simulink model "Non_WindFarm"  (R2024a)
settings: Solver=ode45  StartTime=parSimulacio.ti  StopTime=200  MaxStep=parSimulacio.pas  RelTol=1e-6  AbsTol=1e-6  EnableMultiTasking=on
model workspace (MAT data in the model file):
  tt_vw = Simulink.Parameter
  tt_vw.Complexity = 'real'
  tt_vw.Dimensions = [0 0]
  tt_vw.DataType = 'auto'
values from neighbouring files (symbols this model uses):
  L = L'    [Lin_SignalGenerator.m]    (also in Non_ParameterInitialize.m; cal_QR.m = zeros(v, 1); parameters_windFarm2.m)
  nu = size(S, 1)    [Lin_SignalGenerator.m]    (also in Non_ParameterInitialize.m; parameters_windFarm2.m)
  S = zeros(v, v)    [cal_QR.m]
  w0 = [1 -0.00962521549583 0.0254779042049 -0.0160197396127 -0.0156056332727 0.0112137208272 0.0440607583301 -0.0193704893312 -0.0229464276306 -0.00247675309015 0.0285830611299]    [w0.mat]
undefined symbols (not defined in the file or in its folder): parControl, parConvertidor, parGenerador, parGrid, parMecanica, parSimulacio, windspeed
(part 1 of 40)
settings Model: SimulationMode=accelerator  Creator=adria  LastModifiedBy=hz1021
settings SolverCC: AlgebraicLoopSolver=TrustRegion
settings DataIOCC: LimitDataPoints=on  SaveFormat=Array  SignalLoggingSaveFormat=ModelDataLogs  SaveOutput=off  SaveTime=off  ReturnWorkspaceOutputs=off
settings OptimizationCC: ReuseModelBlockBuffer=off  InitFltsAndDblsToZero=on  LifeSpan=inf
settings DebuggingCC: SaveWithParameterizedLinksMsg=none  UnderspecifiedInitializationDetection=Classic  MergeDetectMultiDrivingBlocksExec=none  SignalResolutionControl=TryResolveAllWithWarning  SolverPrmCheckMsg=warning  FcnCallInpInsideContextMsg=warning  UnconnectedInputMsg=warning  UnconnectedOutputMsg=warning  UnconnectedLineMsg=warning  SFUnexpectedBacktrackingDiag=warning  SFNoUnconditionalDefaultTransitionDiag=warning  SFExecutionAtInitializationDiag=none  ArithmeticOperatorsInVariantConditions=warning
settings HardwareCC: ProdBitPerPointer=32  ProdBitPerSizeT=32  ProdBitPerPtrDiffT=32  ProdLargestAtomicFloat=None  ProdIntDivRoundTo=Undefined  ProdEndianess=Unspecified  ProdWordSize=32  ProdHWDeviceType=32-bit Generic
settings ModelReferenceCC: EnableRefExpFcnMdlSchedulingChecks=on  PropagateSignalLabelsOutOfModel=off
settings RTWCC: GPUComputeCapability=3.5  DLArmComputeVersion=19.05
settings CodeAppCC: StateflowObjectComments=on
settings GRTTargetCC: TargetFcnLib=ansi_tfl_tmw.mat  TargetLangStandard=C89/C90 (ANSI)  CombineOutputUpdateFcns=off  GRTInterface=on
settings ConfigComp: CovMetricSettings=dw  CovSaveCumulativeToWorkspaceVar=on  CovSaveSingleToWorkspaceVar=on

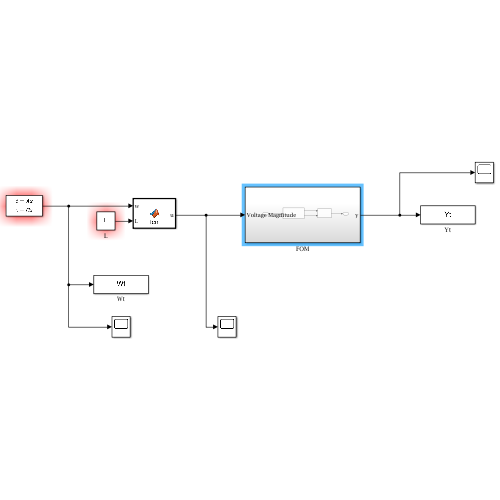
[thumbnail: Simulink's stored preview of the top-level diagram]
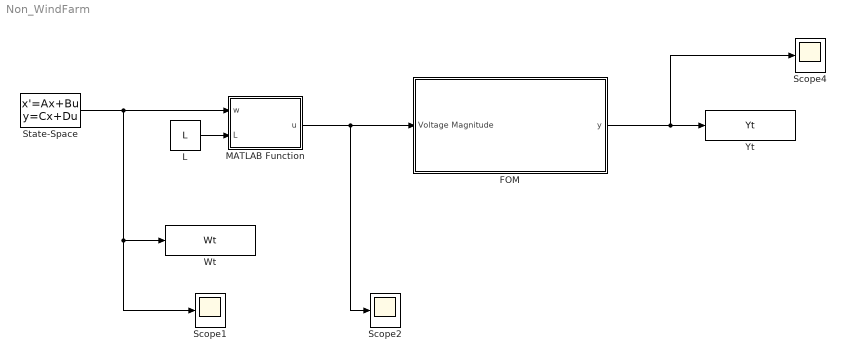
== system Non_WindFarm ==
  FOM : Subsystem
  L : Constant  Value=L
  MATLAB Function : MATLAB Function  TreatAsAtomicUnit=on
  Scope1 : Scope
  Scope2 : Scope
  Scope4 : Scope
  State-Space : StateSpace  A=S  B=[]  C=eye(nu)  D=[]  InitialCondition=w0  AbsoluteTolerance=1e-6
  Wt : ToWorkspace  VariableName=Wt  SaveFormat=Timeseries  SampleTime=-1
  Yt : ToWorkspace  VariableName=Yt  SaveFormat=Timeseries  SampleTime=-1
  wires:
  FOM/1(y) -> Yt/1, Scope4/1
  MATLAB Function/1(u) -> FOM/1(Voltage Magnitude), Scope2/1
  State-Space/1 -> Wt/1, Scope1/1, MATLAB Function/1(w)
  L/1 -> MATLAB Function/2(L)

== system Non_WindFarm/FOM ==
  Voltage Magnitude : Inport
  MATLAB Function2 : MATLAB Function  TreatAsAtomicUnit=on
  Wind Farm : Subsystem
  y : Outport
  wires:
  Wind Farm/2(Ic) -> MATLAB Function2/2(Ic)
  Voltage Magnitude/1 -> Wind Farm/1(Voltage Magnitude)
  Wind Farm/1(Vc) -> MATLAB Function2/1(Vc)
  MATLAB Function2/1(y) -> y/1

== system Non_WindFarm/FOM/Wind Farm ==
  Voltage Magnitude : Inport
  3phase2dq : Subsystem
  C at HV transf : Subsystem
  Gain1 : Gain  Gain=1/parGrid.WFtransf.rloss
  HV transf1 : Subsystem
  Scope1 : Scope
  Scope3 : Scope
  Subtract1 : Sum  Inputs=+-
  Wind Turbine Strings : Subsystem
  Vc : Outport
  Ic : Outport  Port=2
  wires:
  Subtract1/1 -> Scope3/1, Ic/1, C at HV transf/2(Itransf)
  3phase2dq/1(Vdq) -> HV transf1/1(Vin)
  HV transf1/1(Itransf) -> Subtract1/1
  C at HV transf/1(Vc) -> Wind Turbine Strings/1(V_in), Scope1/1, Vc/1, HV transf1/2(Vc), Gain1/1
  Gain1/1 -> Subtract1/2
  Voltage Magnitude/1 -> 3phase2dq/1(Voltage Magnitude)
  Wind Turbine Strings/1(I_out_tol) -> C at HV transf/1(Istrings)

== system Non_WindFarm/FOM/Wind Farm/3phase2dq ==
  Voltage Magnitude : Inport
  Clock2 : Clock
  Font trifasica asimetrica1 : Subsystem  mask{tempPar=parGrid.WFtransf}
      mask prompts: tempPar "Estruc. Parametres"
      mask init:
      | we=tempPar.f*2*pi;
      | A_D=tempPar.V_D*sqrt(2)/sqrt(3);
      | A_I=tempPar.V_I*sqrt(2)/sqrt(3);
      | phi_D=tempPar.phi_D;
      | phi_I=tempPar.phi_I;
      | tt_D=tempPar.tt_D;
      | tt_I=tempPar.tt_I;
      | tA_D=tempPar.tA_D;
      | tA_I=tempPar.tA_I;
  Product : Product
  Vdq : Outport
  wires:
  Product/1 -> Vdq/1
  Clock2/1 -> Font trifasica asimetrica1/1(t)
  Font trifasica asimetrica1/1(y) -> Product/1
  Voltage Magnitude/1 -> Product/2

== system Non_WindFarm/FOM/Wind Farm/C at HV transf ==
  note: Vc_cable
  Istrings : Inport
  Itransf : Inport  Port=2
  Add : Sum  Inputs=+-
  produce Vc_cable : StateSpace  A=[0,-100*pi;100*pi,0]  B=eye(2)/parGrid.WFtransf.Cfilt  C=eye(2)  D=zeros(2,2)  InitialCondition=sqrt(2)*66000/sqrt(3)*[1;0]
  Vc : Outport
  wires:
  produce Vc_cable/1 -> Vc/1
  Add/1 -> produce Vc_cable/1
  Itransf/1 -> Add/2
  Istrings/1 -> Add/1

== system Non_WindFarm/FOM/Wind Farm/HV transf1 ==
  Vin : Inport
  Vc : Inport  Port=2
  1/L_Cable : Gain  Gain=1/parGrid.WFtransf.L
  A : Constant  Value=[parGrid.WFtransf.r,100*pi*parGrid.WFtransf.L;-100*pi*parGrid.WFtransf.L,parGrid.WFtransf.r]
  Add : Sum  Inputs=+--
  Integrator : Integrator
  Product6 : Product  Multiplication=Matrix(*)
  Itransf : Outport
  wires:
  Integrator/1 -> Product6/2, Itransf/1
  Vc/1 -> Add/1
  Vin/1 -> Add/2
  A/1 -> Product6/1
  Product6/1 -> Add/3
  1/L_Cable/1 -> Integrator/1
  Add/1 -> 1/L_Cable/1

== system Non_WindFarm/FOM/Wind Farm/Wind Turbine Strings ==
  V_in : Inport
  Add : Sum  Inputs=6
  String1 : Subsystem
  String2 : Subsystem
  String3 : Subsystem  Commented=on
  String4 : Subsystem  Commented=on
  String5 : Subsystem  Commented=on
  String6 : Subsystem  Commented=on
  I_out_tol : Outport
  wires:
  V_in/1 -> String6/1(V_in), String5/1(V_in), String4/1(V_in), String3/1(V_in), String2/1(V_in), String1/1(V_in)
  String1/1(I_out) -> Add/1
  String2/1(I_out) -> Add/2
  Add/1 -> I_out_tol/1
  String3/1(I_out) -> Add/3
  String4/1(I_out) -> Add/4
  String5/1(I_out) -> Add/5
  String6/1(I_out) -> Add/6

== system Non_WindFarm/FOM/Wind Farm/3phase2dq/Font trifasica asimetrica1 ==
  t : Inport
  Clock : Clock
  Constant1 : Constant  Value=phi_D
  Constant2 : Constant  Value=phi_I
  Constant3 : Constant  Value=2*pi/3
  Constant4 : Constant  Value=2*pi/3
  Gain : Gain  Gain=we
  Gain1 : Gain  Gain=A_D
  Gain2 : Gain  Gain=A_I
  Mux : Mux  Inputs=3
  Mux1 : Mux  Inputs=3
  Park : Subsystem
  Product : Product  RndMeth=Zero
  Product1 : Product  RndMeth=Zero
  Product4 : Product  Multiplication=Matrix(*)  RndMeth=Zero
  Scope1 : Scope
  Sum{1,3,5..7} (5 alike) : Sum  Inputs=|++
  Sum2 : Sum  Inputs=|+-
  Sum4 : Sum  Inputs=|+-
  Trigonometric Function{1..6} (6 alike) : Trigonometry  Operator=cos
  directa : Lookup  InputValues=tt_D  Table=tA_D  SaturateOnIntegerOverflow=off
  inversa : Lookup  InputValues=tt_I  Table=tA_I  SaturateOnIntegerOverflow=off
  we : Gain  Gain=100*pi
  y : Outport
  wires:
  Sum3/1 -> Trigonometric Function2/1, Sum2/1, Sum1/1
  Sum2/1 -> Trigonometric Function1/1
  Sum1/1 -> Trigonometric Function3/1
  Constant4/1 -> Sum2/2, Sum1/2
  Trigonometric Function2/1 -> Mux/1
  Trigonometric Function1/1 -> Mux/2
  Trigonometric Function3/1 -> Mux/3
  Mux/1 -> Gain1/1
  t/1 -> Gain/1, directa/1, inversa/1
  Gain/1 -> Sum3/1, Sum6/1
  Constant1/1 -> Sum3/2
  Sum6/1 -> Trigonometric Function5/1, Sum5/1, Sum4/1
  Sum5/1 -> Trigonometric Function4/1
  Sum4/1 -> Trigonometric Function6/1
  Constant3/1 -> Sum4/2, Sum5/2
  Trigonometric Function5/1 -> Mux1/1
  Trigonometric Function4/1 -> Mux1/2
  Trigonometric Function6/1 -> Mux1/3
  Mux1/1 -> Gain2/1
  Constant2/1 -> Sum6/2
  Product/1 -> Sum7/1
  directa/1 -> Product/1
  inversa/1 -> Product1/1
  Gain1/1 -> Product/2
  Gain2/1 -> Product1/2
  Product1/1 -> Sum7/2
  Park/1(Tthetar) -> Scope1/1, Product4/1
  Clock/1 -> we/1
  we/1 -> Park/1(theta_r)
  Sum7/1 -> Product4/2
  Product4/1 -> y/1

== system Non_WindFarm/FOM/Wind Farm/Wind Turbine Strings/String1 ==
  V_in : Inport
  Constant : Constant  Value=0
  Scope : Scope
  WT1 : Subsystem
  WT10 : Subsystem
  WT2 : Subsystem
  WT3 : Subsystem
  WT4 : Subsystem
  WT5 : Subsystem
  WT6 : Subsystem
  WT7 : Subsystem
  WT8 : Subsystem
  WT9 : Subsystem
  I_out : Outport
  wires:
  WT10/1(V_out) -> Scope/1
  WT7/1(V_out) -> WT8/1(V_in)
  Constant/1 -> WT10/2(I_in)
  WT4/1(V_out) -> WT5/1(V_in)
  WT4/2(I_out) -> WT3/2(I_in)
  WT3/1(V_out) -> WT4/1(V_in)
  WT1/1(V_out) -> WT2/1(V_in)
  WT10/2(I_out) -> WT9/2(I_in)
  WT5/1(V_out) -> WT6/1(V_in)
  WT2/1(V_out) -> WT3/1(V_in)
  WT7/2(I_out) -> WT6/2(I_in)
  WT8/1(V_out) -> WT9/1(V_in)
  WT6/1(V_out) -> WT7/1(V_in)
  WT9/2(I_out) -> WT8/2(I_in)
  WT5/2(I_out) -> WT4/2(I_in)
  WT2/2(I_out) -> WT1/2(I_in)
  V_in/1 -> WT1/1(V_in)
  WT3/2(I_out) -> WT2/2(I_in)
  WT8/2(I_out) -> WT7/2(I_in)
  WT9/1(V_out) -> WT10/1(V_in)
  WT6/2(I_out) -> WT5/2(I_in)
  WT1/2(I_out) -> I_out/1

== system Non_WindFarm/FOM/Wind Farm/Wind Turbine Strings/String2 ==
  V_in : Inport
  Constant : Constant  Value=0
  Scope : Scope
  WT1 : Subsystem
  WT10 : Subsystem
  WT2 : Subsystem
  WT3 : Subsystem
  WT4 : Subsystem
  WT5 : Subsystem
  WT6 : Subsystem
  WT7 : Subsystem
  WT8 : Subsystem
  WT9 : Subsystem
  I_out : Outport
  wires:
  WT1/2(I_out) -> I_out/1
  WT6/2(I_out) -> WT5/2(I_in)
  WT9/1(V_out) -> WT10/1(V_in)
  WT8/2(I_out) -> WT7/2(I_in)
  WT3/2(I_out) -> WT2/2(I_in)
  V_in/1 -> WT1/1(V_in)
  WT2/2(I_out) -> WT1/2(I_in)
  WT5/2(I_out) -> WT4/2(I_in)
  WT9/2(I_out) -> WT8/2(I_in)
  WT6/1(V_out) -> WT7/1(V_in)
  WT8/1(V_out) -> WT9/1(V_in)
  WT7/2(I_out) -> WT6/2(I_in)
  WT2/1(V_out) -> WT3/1(V_in)
  WT5/1(V_out) -> WT6/1(V_in)
  WT10/2(I_out) -> WT9/2(I_in)
  WT1/1(V_out) -> WT2/1(V_in)
  WT3/1(V_out) -> WT4/1(V_in)
  WT4/2(I_out) -> WT3/2(I_in)
  WT4/1(V_out) -> WT5/1(V_in)
  Constant/1 -> WT10/2(I_in)
  WT7/1(V_out) -> WT8/1(V_in)
  WT10/1(V_out) -> Scope/1

== system Non_WindFarm/FOM/Wind Farm/Wind Turbine Strings/String3 ==
  V_in : Inport
  Constant : Constant  Value=0
  Scope : Scope
  WT1 : Subsystem
  WT10 : Subsystem
  WT2 : Subsystem
  WT3 : Subsystem
  WT4 : Subsystem
  WT5 : Subsystem
  WT6 : Subsystem
  WT7 : Subsystem
  WT8 : Subsystem
  WT9 : Subsystem
  I_out : Outport
  wires:
  WT1/2(I_out) -> I_out/1
  WT6/2(I_out) -> WT5/2(I_in)
  WT9/1(V_out) -> WT10/1(V_in)
  WT8/2(I_out) -> WT7/2(I_in)
  WT3/2(I_out) -> WT2/2(I_in)
  V_in/1 -> WT1/1(V_in)
  WT2/2(I_out) -> WT1/2(I_in)
  WT5/2(I_out) -> WT4/2(I_in)
  WT9/2(I_out) -> WT8/2(I_in)
  WT6/1(V_out) -> WT7/1(V_in)
  WT8/1(V_out) -> WT9/1(V_in)
  WT7/2(I_out) -> WT6/2(I_in)
  WT2/1(V_out) -> WT3/1(V_in)
  WT5/1(V_out) -> WT6/1(V_in)
  WT10/2(I_out) -> WT9/2(I_in)
  WT1/1(V_out) -> WT2/1(V_in)
  WT3/1(V_out) -> WT4/1(V_in)
  WT4/2(I_out) -> WT3/2(I_in)
  WT4/1(V_out) -> WT5/1(V_in)
  Constant/1 -> WT10/2(I_in)
  WT7/1(V_out) -> WT8/1(V_in)
  WT10/1(V_out) -> Scope/1

== system Non_WindFarm/FOM/Wind Farm/Wind Turbine Strings/String4 ==
  V_in : Inport
  Constant : Constant  Value=0
  Scope : Scope
  WT1 : Subsystem
  WT10 : Subsystem
  WT2 : Subsystem
  WT3 : Subsystem
  WT4 : Subsystem
  WT5 : Subsystem
  WT6 : Subsystem
  WT7 : Subsystem
  WT8 : Subsystem
  WT9 : Subsystem
  I_out : Outport
  wires:
  WT1/2(I_out) -> I_out/1
  WT6/2(I_out) -> WT5/2(I_in)
  WT9/1(V_out) -> WT10/1(V_in)
  WT8/2(I_out) -> WT7/2(I_in)
  WT3/2(I_out) -> WT2/2(I_in)
  V_in/1 -> WT1/1(V_in)
  WT2/2(I_out) -> WT1/2(I_in)
  WT5/2(I_out) -> WT4/2(I_in)
  WT9/2(I_out) -> WT8/2(I_in)
  WT6/1(V_out) -> WT7/1(V_in)
  WT8/1(V_out) -> WT9/1(V_in)
  WT7/2(I_out) -> WT6/2(I_in)
  WT2/1(V_out) -> WT3/1(V_in)
  WT5/1(V_out) -> WT6/1(V_in)
  WT10/2(I_out) -> WT9/2(I_in)
  WT1/1(V_out) -> WT2/1(V_in)
  WT3/1(V_out) -> WT4/1(V_in)
  WT4/2(I_out) -> WT3/2(I_in)
  WT4/1(V_out) -> WT5/1(V_in)
  Constant/1 -> WT10/2(I_in)
  WT7/1(V_out) -> WT8/1(V_in)
  WT10/1(V_out) -> Scope/1

== system Non_WindFarm/FOM/Wind Farm/Wind Turbine Strings/String5 ==
  V_in : Inport
  Constant : Constant  Value=0
  Scope : Scope
  WT1 : Subsystem
  WT10 : Subsystem
  WT2 : Subsystem
  WT3 : Subsystem
  WT4 : Subsystem
  WT5 : Subsystem
  WT6 : Subsystem
  WT7 : Subsystem
  WT8 : Subsystem
  WT9 : Subsystem
  I_out : Outport
  wires:
  WT1/2(I_out) -> I_out/1
  WT6/2(I_out) -> WT5/2(I_in)
  WT9/1(V_out) -> WT10/1(V_in)
  WT8/2(I_out) -> WT7/2(I_in)
  WT3/2(I_out) -> WT2/2(I_in)
  V_in/1 -> WT1/1(V_in)
  WT2/2(I_out) -> WT1/2(I_in)
  WT5/2(I_out) -> WT4/2(I_in)
  WT9/2(I_out) -> WT8/2(I_in)
  WT6/1(V_out) -> WT7/1(V_in)
  WT8/1(V_out) -> WT9/1(V_in)
  WT7/2(I_out) -> WT6/2(I_in)
  WT2/1(V_out) -> WT3/1(V_in)
  WT5/1(V_out) -> WT6/1(V_in)
  WT10/2(I_out) -> WT9/2(I_in)
  WT1/1(V_out) -> WT2/1(V_in)
  WT3/1(V_out) -> WT4/1(V_in)
  WT4/2(I_out) -> WT3/2(I_in)
  WT4/1(V_out) -> WT5/1(V_in)
  Constant/1 -> WT10/2(I_in)
  WT7/1(V_out) -> WT8/1(V_in)
  WT10/1(V_out) -> Scope/1

== system Non_WindFarm/FOM/Wind Farm/Wind Turbine Strings/String6 ==
  V_in : Inport
  Constant : Constant  Value=0
  Scope : Scope
  WT1 : Subsystem
  WT10 : Subsystem
  WT2 : Subsystem
  WT3 : Subsystem
  WT4 : Subsystem
  WT5 : Subsystem
  WT6 : Subsystem
  WT7 : Subsystem
  WT8 : Subsystem
  WT9 : Subsystem
  I_out : Outport
  wires:
  WT1/2(I_out) -> I_out/1
  WT6/2(I_out) -> WT5/2(I_in)
  WT9/1(V_out) -> WT10/1(V_in)
  WT8/2(I_out) -> WT7/2(I_in)
  WT3/2(I_out) -> WT2/2(I_in)
  V_in/1 -> WT1/1(V_in)
  WT2/2(I_out) -> WT1/2(I_in)
  WT5/2(I_out) -> WT4/2(I_in)
  WT9/2(I_out) -> WT8/2(I_in)
  WT6/1(V_out) -> WT7/1(V_in)
  WT8/1(V_out) -> WT9/1(V_in)
  WT7/2(I_out) -> WT6/2(I_in)
  WT2/1(V_out) -> WT3/1(V_in)
  WT5/1(V_out) -> WT6/1(V_in)
  WT10/2(I_out) -> WT9/2(I_in)
  WT1/1(V_out) -> WT2/1(V_in)
  WT3/1(V_out) -> WT4/1(V_in)
  WT4/2(I_out) -> WT3/2(I_in)
  WT4/1(V_out) -> WT5/1(V_in)
  Constant/1 -> WT10/2(I_in)
  WT7/1(V_out) -> WT8/1(V_in)
  WT10/1(V_out) -> Scope/1

== system Non_WindFarm/FOM/Wind Farm/3phase2dq/Font trifasica asimetrica1/Park ==
  theta_r : Inport
  Constant4 : Constant  Value=2*pi/3
  Gain7 : Gain  Gain=2/3
  Matrix Concatenate1 : Concatenate  NumInputs=3  Mode=Multidimensional array  ConcatenateDimension=2
  Matrix Concatenate2 : Concatenate  Mode=Multidimensional array  ConcatenateDimension=2
  Mux2 : Mux  Inputs=2
  Mux3 : Mux  Inputs=2
  Mux4 : Mux  Inputs=2
  Mux5 : Mux  Inputs=3
  Mux6 : Mux  Inputs=3
  Sum1 : Sum  Inputs=|++
  Sum2 : Sum  Inputs=|+-
  Trigonometric Function : Trigonometry  Operator=cos
  Trigonometric Function1 : Trigonometry
  Trigonometric Function2 : Trigonometry  Operator=cos
  Trigonometric Function3 : Trigonometry
  Trigonometric Function4 : Trigonometry  Operator=cos
  Trigonometric Function5 : Trigonometry
  Tthetar : Outport
  nTthetar : Outport  Port=2
  wires:
  theta_r/1 -> Sum1/1, Sum2/1, Trigonometric Function/1, Trigonometric Function1/1
  Sum2/1 -> Trigonometric Function2/1, Trigonometric Function3/1
  Sum1/1 -> Trigonometric Function4/1, Trigonometric Function5/1
  Constant4/1 -> Sum2/2, Sum1/2
  Trigonometric Function/1 -> Mux2/1, Mux5/1
  Trigonometric Function1/1 -> Mux2/2, Mux6/1
  Trigonometric Function2/1 -> Mux3/1, Mux5/2
  Trigonometric Function3/1 -> Mux3/2, Mux6/2
  Trigonometric Function4/1 -> Mux4/1, Mux5/3
  Trigonometric Function5/1 -> Mux4/2, Mux6/3
  Mux2/1 -> Matrix Concatenate1/1
  Mux3/1 -> Matrix Concatenate1/2
  Mux4/1 -> Matrix Concatenate1/3
  Matrix Concatenate1/1 -> Gain7/1
  Mux5/1 -> Matrix Concatenate2/1
  Mux6/1 -> Matrix Concatenate2/2
  Gain7/1 -> Tthetar/1
  Matrix Concatenate2/1 -> nTthetar/1

== system Non_WindFarm/FOM/Wind Farm/Wind Turbine Strings/String1/WT1 ==
  V_in : Inport
  I_in : Inport  Port=2
  Add1 : Sum  Inputs=+-
  C_cable : Subsystem
  C_filter : Subsystem
  Cable line : Subsystem
  Gain : Gain  Gain=1/parGrid.WTstring.Rparallel_cable
  Transformer-complex : Subsystem
  WFG : Subsystem
  V_out : Outport
  I_out : Outport  Port=2
  wires:
  C_cable/1(Vc_cable) -> Gain/1, Transformer-complex/2(Vc_cable_qd), V_out/1, Cable line/2(Vc_cable)
  WFG/1(ilqd) -> C_filter/1(IWF)
  C_filter/1(Vc_filter_qd) -> Transformer-complex/1(Vc_filter_qd), WFG/1(vcqd)
  Cable line/1(I_cable) -> I_out/1, C_cable/3(I_cable)
  Transformer-complex/1(It1) -> C_filter/2(It1)
  V_in/1 -> Cable line/1(V)
  Transformer-complex/2(It2) -> Add1/1
  Add1/1 -> C_cable/1(It2)
  Gain/1 -> Add1/2
  I_in/1 -> C_cable/2(I_in)

== system Non_WindFarm/FOM/Wind Farm/Wind Turbine Strings/String1/WT10 ==
  V_in : Inport
  I_in : Inport  Port=2
  Add1 : Sum  Inputs=+-
  C_cable : Subsystem
  C_filter : Subsystem
  Cable line : Subsystem
  Gain : Gain  Gain=1/parGrid.WTstring.Rparallel_cable
  Transformer-complex : Subsystem
  WFG : Subsystem
  V_out : Outport
  I_out : Outport  Port=2
  wires:
  I_in/1 -> C_cable/2(I_in)
  Gain/1 -> Add1/2
  Add1/1 -> C_cable/1(It2)
  Transformer-complex/2(It2) -> Add1/1
  V_in/1 -> Cable line/1(V)
  Transformer-complex/1(It1) -> C_filter/2(It1)
  Cable line/1(I_cable) -> C_cable/3(I_cable), I_out/1
  C_filter/1(Vc_filter_qd) -> WFG/1(vcqd), Transformer-complex/1(Vc_filter_qd)
  WFG/1(ilqd) -> C_filter/1(IWF)
  C_cable/1(Vc_cable) -> Cable line/2(Vc_cable), V_out/1, Transformer-complex/2(Vc_cable_qd), Gain/1

== system Non_WindFarm/FOM/Wind Farm/Wind Turbine Strings/String1/WT2 ==
  V_in : Inport
  I_in : Inport  Port=2
  Add1 : Sum  Inputs=+-
  C_cable : Subsystem
  C_filter : Subsystem
  Cable line : Subsystem
  Gain : Gain  Gain=1/parGrid.WTstring.Rparallel_cable
  Transformer-complex : Subsystem
  WFG : Subsystem
  V_out : Outport
  I_out : Outport  Port=2
  wires:
  I_in/1 -> C_cable/2(I_in)
  Gain/1 -> Add1/2
  Add1/1 -> C_cable/1(It2)
  Transformer-complex/2(It2) -> Add1/1
  V_in/1 -> Cable line/1(V)
  Transformer-complex/1(It1) -> C_filter/2(It1)
  Cable line/1(I_cable) -> C_cable/3(I_cable), I_out/1
  C_filter/1(Vc_filter_qd) -> WFG/1(vcqd), Transformer-complex/1(Vc_filter_qd)
  WFG/1(ilqd) -> C_filter/1(IWF)
  C_cable/1(Vc_cable) -> Cable line/2(Vc_cable), V_out/1, Transformer-complex/2(Vc_cable_qd), Gain/1

== system Non_WindFarm/FOM/Wind Farm/Wind Turbine Strings/String1/WT3 ==
  V_in : Inport
  I_in : Inport  Port=2
  Add1 : Sum  Inputs=+-
  C_cable : Subsystem
  C_filter : Subsystem
  Cable line : Subsystem
  Gain : Gain  Gain=1/parGrid.WTstring.Rparallel_cable
  Transformer-complex : Subsystem
  WFG : Subsystem
  V_out : Outport
  I_out : Outport  Port=2
  wires:
  C_cable/1(Vc_cable) -> Gain/1, Transformer-complex/2(Vc_cable_qd), V_out/1, Cable line/2(Vc_cable)
  WFG/1(ilqd) -> C_filter/1(IWF)
  C_filter/1(Vc_filter_qd) -> WFG/1(vcqd), Transformer-complex/1(Vc_filter_qd)
  Cable line/1(I_cable) -> I_out/1, C_cable/3(I_cable)
  Transformer-complex/1(It1) -> C_filter/2(It1)
  V_in/1 -> Cable line/1(V)
  Transformer-complex/2(It2) -> Add1/1
  Add1/1 -> C_cable/1(It2)
  Gain/1 -> Add1/2
  I_in/1 -> C_cable/2(I_in)

== system Non_WindFarm/FOM/Wind Farm/Wind Turbine Strings/String1/WT4 ==
  V_in : Inport
  I_in : Inport  Port=2
  Add1 : Sum  Inputs=+-
  C_cable : Subsystem
  C_filter : Subsystem
  Cable line : Subsystem
  Gain : Gain  Gain=1/parGrid.WTstring.Rparallel_cable
  Transformer-complex : Subsystem
  WFG : Subsystem
  V_out : Outport
  I_out : Outport  Port=2
  wires:
  I_in/1 -> C_cable/2(I_in)
  Gain/1 -> Add1/2
  Add1/1 -> C_cable/1(It2)
  Transformer-complex/2(It2) -> Add1/1
  V_in/1 -> Cable line/1(V)
  Transformer-complex/1(It1) -> C_filter/2(It1)
  Cable line/1(I_cable) -> C_cable/3(I_cable), I_out/1
  C_filter/1(Vc_filter_qd) -> WFG/1(vcqd), Transformer-complex/1(Vc_filter_qd)
  WFG/1(ilqd) -> C_filter/1(IWF)
  C_cable/1(Vc_cable) -> Cable line/2(Vc_cable), V_out/1, Transformer-complex/2(Vc_cable_qd), Gain/1

== system Non_WindFarm/FOM/Wind Farm/Wind Turbine Strings/String1/WT5 ==
  V_in : Inport
  I_in : Inport  Port=2
  Add1 : Sum  Inputs=+-
  C_cable : Subsystem
  C_filter : Subsystem
  Cable line : Subsystem
  Gain : Gain  Gain=1/parGrid.WTstring.Rparallel_cable
  Transformer-complex : Subsystem
  WFG : Subsystem
  V_out : Outport
  I_out : Outport  Port=2
  wires:
  C_cable/1(Vc_cable) -> Gain/1, Transformer-complex/2(Vc_cable_qd), V_out/1, Cable line/2(Vc_cable)
  WFG/1(ilqd) -> C_filter/1(IWF)
  C_filter/1(Vc_filter_qd) -> WFG/1(vcqd), Transformer-complex/1(Vc_filter_qd)
  Cable line/1(I_cable) -> I_out/1, C_cable/3(I_cable)
  Transformer-complex/1(It1) -> C_filter/2(It1)
  V_in/1 -> Cable line/1(V)
  Transformer-complex/2(It2) -> Add1/1
  Add1/1 -> C_cable/1(It2)
  Gain/1 -> Add1/2
  I_in/1 -> C_cable/2(I_in)

== system Non_WindFarm/FOM/Wind Farm/Wind Turbine Strings/String1/WT6 ==
  V_in : Inport
  I_in : Inport  Port=2
  Add1 : Sum  Inputs=+-
  C_cable : Subsystem
  C_filter : Subsystem
  Cable line : Subsystem
  Gain : Gain  Gain=1/parGrid.WTstring.Rparallel_cable
  Transformer-complex : Subsystem
  WFG : Subsystem
  V_out : Outport
  I_out : Outport  Port=2
  wires:
  I_in/1 -> C_cable/2(I_in)
  Gain/1 -> Add1/2
  Add1/1 -> C_cable/1(It2)
  Transformer-complex/2(It2) -> Add1/1
  V_in/1 -> Cable line/1(V)
  Transformer-complex/1(It1) -> C_filter/2(It1)
  Cable line/1(I_cable) -> C_cable/3(I_cable), I_out/1
  C_filter/1(Vc_filter_qd) -> WFG/1(vcqd), Transformer-complex/1(Vc_filter_qd)
  WFG/1(ilqd) -> C_filter/1(IWF)
  C_cable/1(Vc_cable) -> Cable line/2(Vc_cable), V_out/1, Transformer-complex/2(Vc_cable_qd), Gain/1

== system Non_WindFarm/FOM/Wind Farm/Wind Turbine Strings/String1/WT7 ==
  V_in : Inport
  I_in : Inport  Port=2
  Add1 : Sum  Inputs=+-
  C_cable : Subsystem
  C_filter : Subsystem
  Cable line : Subsystem
  Gain : Gain  Gain=1/parGrid.WTstring.Rparallel_cable
  Transformer-complex : Subsystem
  WFG : Subsystem
  V_out : Outport
  I_out : Outport  Port=2
  wires:
  C_cable/1(Vc_cable) -> Gain/1, Transformer-complex/2(Vc_cable_qd), V_out/1, Cable line/2(Vc_cable)
  WFG/1(ilqd) -> C_filter/1(IWF)
  C_filter/1(Vc_filter_qd) -> WFG/1(vcqd), Transformer-complex/1(Vc_filter_qd)
  Cable line/1(I_cable) -> I_out/1, C_cable/3(I_cable)
  Transformer-complex/1(It1) -> C_filter/2(It1)
  V_in/1 -> Cable line/1(V)
  Transformer-complex/2(It2) -> Add1/1
  Add1/1 -> C_cable/1(It2)
  Gain/1 -> Add1/2
  I_in/1 -> C_cable/2(I_in)

== system Non_WindFarm/FOM/Wind Farm/Wind Turbine Strings/String1/WT8 ==
  V_in : Inport
  I_in : Inport  Port=2
  Add1 : Sum  Inputs=+-
  C_cable : Subsystem
  C_filter : Subsystem
  Cable line : Subsystem
  Gain : Gain  Gain=1/parGrid.WTstring.Rparallel_cable
  Transformer-complex : Subsystem
  WFG : Subsystem
  V_out : Outport
  I_out : Outport  Port=2
  wires:
  I_in/1 -> C_cable/2(I_in)
  Gain/1 -> Add1/2
  Add1/1 -> C_cable/1(It2)
  Transformer-complex/2(It2) -> Add1/1
  V_in/1 -> Cable line/1(V)
  Transformer-complex/1(It1) -> C_filter/2(It1)
  Cable line/1(I_cable) -> C_cable/3(I_cable), I_out/1
  C_filter/1(Vc_filter_qd) -> WFG/1(vcqd), Transformer-complex/1(Vc_filter_qd)
  WFG/1(ilqd) -> C_filter/1(IWF)
  C_cable/1(Vc_cable) -> Cable line/2(Vc_cable), V_out/1, Transformer-complex/2(Vc_cable_qd), Gain/1

== system Non_WindFarm/FOM/Wind Farm/Wind Turbine Strings/String1/WT9 ==
  V_in : Inport
  I_in : Inport  Port=2
  Add1 : Sum  Inputs=+-
  C_cable : Subsystem
  C_filter : Subsystem
  Cable line : Subsystem
  Gain : Gain  Gain=1/parGrid.WTstring.Rparallel_cable
  Transformer-complex : Subsystem
  WFG : Subsystem
  V_out : Outport
  I_out : Outport  Port=2
  wires:
  C_cable/1(Vc_cable) -> Gain/1, Transformer-complex/2(Vc_cable_qd), V_out/1, Cable line/2(Vc_cable)
  WFG/1(ilqd) -> C_filter/1(IWF)
  C_filter/1(Vc_filter_qd) -> WFG/1(vcqd), Transformer-complex/1(Vc_filter_qd)
  Cable line/1(I_cable) -> I_out/1, C_cable/3(I_cable)
  Transformer-complex/1(It1) -> C_filter/2(It1)
  V_in/1 -> Cable line/1(V)
  Transformer-complex/2(It2) -> Add1/1
  Add1/1 -> C_cable/1(It2)
  Gain/1 -> Add1/2
  I_in/1 -> C_cable/2(I_in)

== system Non_WindFarm/FOM/Wind Farm/Wind Turbine Strings/String2/WT1 ==
  V_in : Inport
  I_in : Inport  Port=2
  Add1 : Sum  Inputs=+-
  C_cable : Subsystem
  C_filter : Subsystem
  Cable line : Subsystem
  Gain : Gain  Gain=1/parGrid.WTstring.Rparallel_cable
  Transformer-complex : Subsystem
  WFG : Subsystem
  V_out : Outport
  I_out : Outport  Port=2
  wires:
  I_in/1 -> C_cable/2(I_in)
  Gain/1 -> Add1/2
  Add1/1 -> C_cable/1(It2)
  Transformer-complex/2(It2) -> Add1/1
  V_in/1 -> Cable line/1(V)
  Transformer-complex/1(It1) -> C_filter/2(It1)
  Cable line/1(I_cable) -> C_cable/3(I_cable), I_out/1
  C_filter/1(Vc_filter_qd) -> WFG/1(vcqd), Transformer-complex/1(Vc_filter_qd)
  WFG/1(ilqd) -> C_filter/1(IWF)
  C_cable/1(Vc_cable) -> Cable line/2(Vc_cable), V_out/1, Transformer-complex/2(Vc_cable_qd), Gain/1

== system Non_WindFarm/FOM/Wind Farm/Wind Turbine Strings/String2/WT10 ==
  V_in : Inport
  I_in : Inport  Port=2
  Add1 : Sum  Inputs=+-
  C_cable : Subsystem
  C_filter : Subsystem
  Cable line : Subsystem
  Gain : Gain  Gain=1/parGrid.WTstring.Rparallel_cable
  Transformer-complex : Subsystem
  WFG : Subsystem
  V_out : Outport
  I_out : Outport  Port=2
  wires:
  C_cable/1(Vc_cable) -> Gain/1, Transformer-complex/2(Vc_cable_qd), V_out/1, Cable line/2(Vc_cable)
  WFG/1(ilqd) -> C_filter/1(IWF)
  C_filter/1(Vc_filter_qd) -> Transformer-complex/1(Vc_filter_qd), WFG/1(vcqd)
  Cable line/1(I_cable) -> I_out/1, C_cable/3(I_cable)
  Transformer-complex/1(It1) -> C_filter/2(It1)
  V_in/1 -> Cable line/1(V)
  Transformer-complex/2(It2) -> Add1/1
  Add1/1 -> C_cable/1(It2)
  Gain/1 -> Add1/2
  I_in/1 -> C_cable/2(I_in)

== system Non_WindFarm/FOM/Wind Farm/Wind Turbine Strings/String2/WT2 ==
  V_in : Inport
  I_in : Inport  Port=2
  Add1 : Sum  Inputs=+-
  C_cable : Subsystem
  C_filter : Subsystem
  Cable line : Subsystem
  Gain : Gain  Gain=1/parGrid.WTstring.Rparallel_cable
  Transformer-complex : Subsystem
  WFG : Subsystem
  V_out : Outport
  I_out : Outport  Port=2
  wires:
  C_cable/1(Vc_cable) -> Gain/1, Transformer-complex/2(Vc_cable_qd), V_out/1, Cable line/2(Vc_cable)
  WFG/1(ilqd) -> C_filter/1(IWF)
  C_filter/1(Vc_filter_qd) -> Transformer-complex/1(Vc_filter_qd), WFG/1(vcqd)
  Cable line/1(I_cable) -> I_out/1, C_cable/3(I_cable)
  Transformer-complex/1(It1) -> C_filter/2(It1)
  V_in/1 -> Cable line/1(V)
  Transformer-complex/2(It2) -> Add1/1
  Add1/1 -> C_cable/1(It2)
  Gain/1 -> Add1/2
  I_in/1 -> C_cable/2(I_in)

== system Non_WindFarm/FOM/Wind Farm/Wind Turbine Strings/String2/WT3 ==
  V_in : Inport
  I_in : Inport  Port=2
  Add1 : Sum  Inputs=+-
  C_cable : Subsystem
  C_filter : Subsystem
  Cable line : Subsystem
  Gain : Gain  Gain=1/parGrid.WTstring.Rparallel_cable
  Transformer-complex : Subsystem
  WFG : Subsystem
  V_out : Outport
  I_out : Outport  Port=2
  wires:
  I_in/1 -> C_cable/2(I_in)
  Gain/1 -> Add1/2
  Add1/1 -> C_cable/1(It2)
  Transformer-complex/2(It2) -> Add1/1
  V_in/1 -> Cable line/1(V)
  Transformer-complex/1(It1) -> C_filter/2(It1)
  Cable line/1(I_cable) -> C_cable/3(I_cable), I_out/1
  C_filter/1(Vc_filter_qd) -> Transformer-complex/1(Vc_filter_qd), WFG/1(vcqd)
  WFG/1(ilqd) -> C_filter/1(IWF)
  C_cable/1(Vc_cable) -> Cable line/2(Vc_cable), V_out/1, Transformer-complex/2(Vc_cable_qd), Gain/1

== system Non_WindFarm/FOM/Wind Farm/Wind Turbine Strings/String2/WT4 ==
  V_in : Inport
  I_in : Inport  Port=2
  Add1 : Sum  Inputs=+-
  C_cable : Subsystem
  C_filter : Subsystem
  Cable line : Subsystem
  Gain : Gain  Gain=1/parGrid.WTstring.Rparallel_cable
  Transformer-complex : Subsystem
  WFG : Subsystem
  V_out : Outport
  I_out : Outport  Port=2
  wires:
  C_cable/1(Vc_cable) -> Gain/1, Transformer-complex/2(Vc_cable_qd), V_out/1, Cable line/2(Vc_cable)
  WFG/1(ilqd) -> C_filter/1(IWF)
  C_filter/1(Vc_filter_qd) -> Transformer-complex/1(Vc_filter_qd), WFG/1(vcqd)
  Cable line/1(I_cable) -> I_out/1, C_cable/3(I_cable)
  Transformer-complex/1(It1) -> C_filter/2(It1)
  V_in/1 -> Cable line/1(V)
  Transformer-complex/2(It2) -> Add1/1
  Add1/1 -> C_cable/1(It2)
  Gain/1 -> Add1/2
  I_in/1 -> C_cable/2(I_in)

== system Non_WindFarm/FOM/Wind Farm/Wind Turbine Strings/String2/WT5 ==
  V_in : Inport
  I_in : Inport  Port=2
  Add1 : Sum  Inputs=+-
  C_cable : Subsystem
  C_filter : Subsystem
  Cable line : Subsystem
  Gain : Gain  Gain=1/parGrid.WTstring.Rparallel_cable
  Transformer-complex : Subsystem
  WFG : Subsystem
  V_out : Outport
  I_out : Outport  Port=2
  wires:
  I_in/1 -> C_cable/2(I_in)
  Gain/1 -> Add1/2
  Add1/1 -> C_cable/1(It2)
  Transformer-complex/2(It2) -> Add1/1
  V_in/1 -> Cable line/1(V)
  Transformer-complex/1(It1) -> C_filter/2(It1)
  Cable line/1(I_cable) -> C_cable/3(I_cable), I_out/1
  C_filter/1(Vc_filter_qd) -> Transformer-complex/1(Vc_filter_qd), WFG/1(vcqd)
  WFG/1(ilqd) -> C_filter/1(IWF)
  C_cable/1(Vc_cable) -> Cable line/2(Vc_cable), V_out/1, Transformer-complex/2(Vc_cable_qd), Gain/1

== system Non_WindFarm/FOM/Wind Farm/Wind Turbine Strings/String2/WT6 ==
  V_in : Inport
  I_in : Inport  Port=2
  Add1 : Sum  Inputs=+-
  C_cable : Subsystem
  C_filter : Subsystem
  Cable line : Subsystem
  Gain : Gain  Gain=1/parGrid.WTstring.Rparallel_cable
  Transformer-complex : Subsystem
  WFG : Subsystem
  V_out : Outport
  I_out : Outport  Port=2
  wires:
  C_cable/1(Vc_cable) -> Gain/1, Transformer-complex/2(Vc_cable_qd), V_out/1, Cable line/2(Vc_cable)
  WFG/1(ilqd) -> C_filter/1(IWF)
  C_filter/1(Vc_filter_qd) -> Transformer-complex/1(Vc_filter_qd), WFG/1(vcqd)
  Cable line/1(I_cable) -> I_out/1, C_cable/3(I_cable)
  Transformer-complex/1(It1) -> C_filter/2(It1)
  V_in/1 -> Cable line/1(V)
  Transformer-complex/2(It2) -> Add1/1
  Add1/1 -> C_cable/1(It2)
  Gain/1 -> Add1/2
  I_in/1 -> C_cable/2(I_in)

== system Non_WindFarm/FOM/Wind Farm/Wind Turbine Strings/String2/WT7 ==
  V_in : Inport
  I_in : Inport  Port=2
  Add1 : Sum  Inputs=+-
  C_cable : Subsystem
  C_filter : Subsystem
  Cable line : Subsystem
  Gain : Gain  Gain=1/parGrid.WTstring.Rparallel_cable
  Transformer-complex : Subsystem
  WFG : Subsystem
  V_out : Outport
  I_out : Outport  Port=2
  wires:
  I_in/1 -> C_cable/2(I_in)
  Gain/1 -> Add1/2
  Add1/1 -> C_cable/1(It2)
  Transformer-complex/2(It2) -> Add1/1
  V_in/1 -> Cable line/1(V)
  Transformer-complex/1(It1) -> C_filter/2(It1)
  Cable line/1(I_cable) -> C_cable/3(I_cable), I_out/1
  C_filter/1(Vc_filter_qd) -> Transformer-complex/1(Vc_filter_qd), WFG/1(vcqd)
  WFG/1(ilqd) -> C_filter/1(IWF)
  C_cable/1(Vc_cable) -> Cable line/2(Vc_cable), V_out/1, Transformer-complex/2(Vc_cable_qd), Gain/1

== system Non_WindFarm/FOM/Wind Farm/Wind Turbine Strings/String2/WT8 ==
  V_in : Inport
  I_in : Inport  Port=2
  Add1 : Sum  Inputs=+-
  C_cable : Subsystem
  C_filter : Subsystem
  Cable line : Subsystem
  Gain : Gain  Gain=1/parGrid.WTstring.Rparallel_cable
  Transformer-complex : Subsystem
  WFG : Subsystem
  V_out : Outport
  I_out : Outport  Port=2
  wires:
  C_cable/1(Vc_cable) -> Gain/1, Transformer-complex/2(Vc_cable_qd), V_out/1, Cable line/2(Vc_cable)
  WFG/1(ilqd) -> C_filter/1(IWF)
  C_filter/1(Vc_filter_qd) -> Transformer-complex/1(Vc_filter_qd), WFG/1(vcqd)
  Cable line/1(I_cable) -> I_out/1, C_cable/3(I_cable)
  Transformer-complex/1(It1) -> C_filter/2(It1)
  V_in/1 -> Cable line/1(V)
  Transformer-complex/2(It2) -> Add1/1
  Add1/1 -> C_cable/1(It2)
  Gain/1 -> Add1/2
  I_in/1 -> C_cable/2(I_in)

== system Non_WindFarm/FOM/Wind Farm/Wind Turbine Strings/String2/WT9 ==
  V_in : Inport
  I_in : Inport  Port=2
  Add1 : Sum  Inputs=+-
  C_cable : Subsystem
  C_filter : Subsystem
  Cable line : Subsystem
  Gain : Gain  Gain=1/parGrid.WTstring.Rparallel_cable
  Transformer-complex : Subsystem
  WFG : Subsystem
  V_out : Outport
  I_out : Outport  Port=2
  wires:
  I_in/1 -> C_cable/2(I_in)
  Gain/1 -> Add1/2
  Add1/1 -> C_cable/1(It2)
  Transformer-complex/2(It2) -> Add1/1
  V_in/1 -> Cable line/1(V)
  Transformer-complex/1(It1) -> C_filter/2(It1)
  Cable line/1(I_cable) -> C_cable/3(I_cable), I_out/1
  C_filter/1(Vc_filter_qd) -> Transformer-complex/1(Vc_filter_qd), WFG/1(vcqd)
  WFG/1(ilqd) -> C_filter/1(IWF)
  C_cable/1(Vc_cable) -> Cable line/2(Vc_cable), V_out/1, Transformer-complex/2(Vc_cable_qd), Gain/1

== system Non_WindFarm/FOM/Wind Farm/Wind Turbine Strings/String3/WT1 ==
  V_in : Inport
  I_in : Inport  Port=2
  Add1 : Sum  Inputs=+-
  C_cable : Subsystem
  C_filter : Subsystem
  Cable line : Subsystem
  Gain : Gain  Gain=1/parGrid.WTstring.Rparallel_cable
  Transformer-complex : Subsystem
  WFG : Subsystem
  V_out : Outport
  I_out : Outport  Port=2
  wires:
  I_in/1 -> C_cable/2(I_in)
  Gain/1 -> Add1/2
  Add1/1 -> C_cable/1(It2)
  Transformer-complex/2(It2) -> Add1/1
  V_in/1 -> Cable line/1(V)
  Transformer-complex/1(It1) -> C_filter/2(It1)
  Cable line/1(I_cable) -> C_cable/3(I_cable), I_out/1
  C_filter/1(Vc_filter_qd) -> WFG/1(vcqd), Transformer-complex/1(Vc_filter_qd)
  WFG/1(ilqd) -> C_filter/1(IWF)
  C_cable/1(Vc_cable) -> Cable line/2(Vc_cable), V_out/1, Transformer-complex/2(Vc_cable_qd), Gain/1

== system Non_WindFarm/FOM/Wind Farm/Wind Turbine Strings/String3/WT10 ==
  V_in : Inport
  I_in : Inport  Port=2
  Add1 : Sum  Inputs=+-
  C_cable : Subsystem
  C_filter : Subsystem
  Cable line : Subsystem
  Gain : Gain  Gain=1/parGrid.WTstring.Rparallel_cable
  Transformer-complex : Subsystem
  WFG : Subsystem
  V_out : Outport
  I_out : Outport  Port=2
  wires:
  C_cable/1(Vc_cable) -> Gain/1, Transformer-complex/2(Vc_cable_qd), V_out/1, Cable line/2(Vc_cable)
  WFG/1(ilqd) -> C_filter/1(IWF)
  C_filter/1(Vc_filter_qd) -> Transformer-complex/1(Vc_filter_qd), WFG/1(vcqd)
  Cable line/1(I_cable) -> I_out/1, C_cable/3(I_cable)
  Transformer-complex/1(It1) -> C_filter/2(It1)
  V_in/1 -> Cable line/1(V)
  Transformer-complex/2(It2) -> Add1/1
  Add1/1 -> C_cable/1(It2)
  Gain/1 -> Add1/2
  I_in/1 -> C_cable/2(I_in)

== system Non_WindFarm/FOM/Wind Farm/Wind Turbine Strings/String3/WT2 ==
  V_in : Inport
  I_in : Inport  Port=2
  Add1 : Sum  Inputs=+-
  C_cable : Subsystem
  C_filter : Subsystem
  Cable line : Subsystem
  Gain : Gain  Gain=1/parGrid.WTstring.Rparallel_cable
  Transformer-complex : Subsystem
  WFG : Subsystem
  V_out : Outport
  I_out : Outport  Port=2
  wires:
  C_cable/1(Vc_cable) -> Gain/1, Transformer-complex/2(Vc_cable_qd), V_out/1, Cable line/2(Vc_cable)
  WFG/1(ilqd) -> C_filter/1(IWF)
  C_filter/1(Vc_filter_qd) -> Transformer-complex/1(Vc_filter_qd), WFG/1(vcqd)
  Cable line/1(I_cable) -> I_out/1, C_cable/3(I_cable)
  Transformer-complex/1(It1) -> C_filter/2(It1)
  V_in/1 -> Cable line/1(V)
  Transformer-complex/2(It2) -> Add1/1
  Add1/1 -> C_cable/1(It2)
  Gain/1 -> Add1/2
  I_in/1 -> C_cable/2(I_in)

== system Non_WindFarm/FOM/Wind Farm/Wind Turbine Strings/String3/WT3 ==
  V_in : Inport
  I_in : Inport  Port=2
  Add1 : Sum  Inputs=+-
  C_cable : Subsystem
  C_filter : Subsystem
  Cable line : Subsystem
  Gain : Gain  Gain=1/parGrid.WTstring.Rparallel_cable
  Transformer-complex : Subsystem
  WFG : Subsystem
  V_out : Outport
  I_out : Outport  Port=2
  wires:
  I_in/1 -> C_cable/2(I_in)
  Gain/1 -> Add1/2
  Add1/1 -> C_cable/1(It2)
  Transformer-complex/2(It2) -> Add1/1
  V_in/1 -> Cable line/1(V)
  Transformer-complex/1(It1) -> C_filter/2(It1)
  Cable line/1(I_cable) -> C_cable/3(I_cable), I_out/1
  C_filter/1(Vc_filter_qd) -> Transformer-complex/1(Vc_filter_qd), WFG/1(vcqd)
  WFG/1(ilqd) -> C_filter/1(IWF)
  C_cable/1(Vc_cable) -> Cable line/2(Vc_cable), V_out/1, Transformer-complex/2(Vc_cable_qd), Gain/1

== system Non_WindFarm/FOM/Wind Farm/Wind Turbine Strings/String3/WT4 ==
  V_in : Inport
  I_in : Inport  Port=2
  Add1 : Sum  Inputs=+-
  C_cable : Subsystem
  C_filter : Subsystem
  Cable line : Subsystem
  Gain : Gain  Gain=1/parGrid.WTstring.Rparallel_cable
  Transformer-complex : Subsystem
  WFG : Subsystem
  V_out : Outport
  I_out : Outport  Port=2
  wires:
  C_cable/1(Vc_cable) -> Gain/1, Transformer-complex/2(Vc_cable_qd), V_out/1, Cable line/2(Vc_cable)
  WFG/1(ilqd) -> C_filter/1(IWF)
  C_filter/1(Vc_filter_qd) -> Transformer-complex/1(Vc_filter_qd), WFG/1(vcqd)
  Cable line/1(I_cable) -> I_out/1, C_cable/3(I_cable)
  Transformer-complex/1(It1) -> C_filter/2(It1)
  V_in/1 -> Cable line/1(V)
  Transformer-complex/2(It2) -> Add1/1
  Add1/1 -> C_cable/1(It2)
  Gain/1 -> Add1/2
  I_in/1 -> C_cable/2(I_in)

== system Non_WindFarm/FOM/Wind Farm/Wind Turbine Strings/String3/WT5 ==
  V_in : Inport
  I_in : Inport  Port=2
  Add1 : Sum  Inputs=+-
  C_cable : Subsystem
  C_filter : Subsystem
  Cable line : Subsystem
  Gain : Gain  Gain=1/parGrid.WTstring.Rparallel_cable
  Transformer-complex : Subsystem
  WFG : Subsystem
  V_out : Outport
  I_out : Outport  Port=2
  wires:
  I_in/1 -> C_cable/2(I_in)
  Gain/1 -> Add1/2
  Add1/1 -> C_cable/1(It2)
  Transformer-complex/2(It2) -> Add1/1
  V_in/1 -> Cable line/1(V)
  Transformer-complex/1(It1) -> C_filter/2(It1)
  Cable line/1(I_cable) -> C_cable/3(I_cable), I_out/1
  C_filter/1(Vc_filter_qd) -> Transformer-complex/1(Vc_filter_qd), WFG/1(vcqd)
  WFG/1(ilqd) -> C_filter/1(IWF)
  C_cable/1(Vc_cable) -> Cable line/2(Vc_cable), V_out/1, Transformer-complex/2(Vc_cable_qd), Gain/1

== system Non_WindFarm/FOM/Wind Farm/Wind Turbine Strings/String3/WT6 ==
  V_in : Inport
  I_in : Inport  Port=2
  Add1 : Sum  Inputs=+-
  C_cable : Subsystem
  C_filter : Subsystem
  Cable line : Subsystem
  Gain : Gain  Gain=1/parGrid.WTstring.Rparallel_cable
  Transformer-complex : Subsystem
  WFG : Subsystem
  V_out : Outport
  I_out : Outport  Port=2
  wires:
  C_cable/1(Vc_cable) -> Gain/1, Transformer-complex/2(Vc_cable_qd), V_out/1, Cable line/2(Vc_cable)
  WFG/1(ilqd) -> C_filter/1(IWF)
  C_filter/1(Vc_filter_qd) -> Transformer-complex/1(Vc_filter_qd), WFG/1(vcqd)
  Cable line/1(I_cable) -> I_out/1, C_cable/3(I_cable)
  Transformer-complex/1(It1) -> C_filter/2(It1)
  V_in/1 -> Cable line/1(V)
  Transformer-complex/2(It2) -> Add1/1
  Add1/1 -> C_cable/1(It2)
  Gain/1 -> Add1/2
  I_in/1 -> C_cable/2(I_in)

== system Non_WindFarm/FOM/Wind Farm/Wind Turbine Strings/String3/WT7 ==
  V_in : Inport
  I_in : Inport  Port=2
  Add1 : Sum  Inputs=+-
  C_cable : Subsystem
  C_filter : Subsystem
  Cable line : Subsystem
  Gain : Gain  Gain=1/parGrid.WTstring.Rparallel_cable
  Transformer-complex : Subsystem
  WFG : Subsystem
  V_out : Outport
  I_out : Outport  Port=2
  wires:
  I_in/1 -> C_cable/2(I_in)
  Gain/1 -> Add1/2
  Add1/1 -> C_cable/1(It2)
  Transformer-complex/2(It2) -> Add1/1
  V_in/1 -> Cable line/1(V)
  Transformer-complex/1(It1) -> C_filter/2(It1)
  Cable line/1(I_cable) -> C_cable/3(I_cable), I_out/1
  C_filter/1(Vc_filter_qd) -> Transformer-complex/1(Vc_filter_qd), WFG/1(vcqd)
  WFG/1(ilqd) -> C_filter/1(IWF)
  C_cable/1(Vc_cable) -> Cable line/2(Vc_cable), V_out/1, Transformer-complex/2(Vc_cable_qd), Gain/1

== system Non_WindFarm/FOM/Wind Farm/Wind Turbine Strings/String3/WT8 ==
  V_in : Inport
  I_in : Inport  Port=2
  Add1 : Sum  Inputs=+-
  C_cable : Subsystem
  C_filter : Subsystem
  Cable line : Subsystem
  Gain : Gain  Gain=1/parGrid.WTstring.Rparallel_cable
  Transformer-complex : Subsystem
  WFG : Subsystem
  V_out : Outport
  I_out : Outport  Port=2
  wires:
  C_cable/1(Vc_cable) -> Gain/1, Transformer-complex/2(Vc_cable_qd), V_out/1, Cable line/2(Vc_cable)
  WFG/1(ilqd) -> C_filter/1(IWF)
  C_filter/1(Vc_filter_qd) -> Transformer-complex/1(Vc_filter_qd), WFG/1(vcqd)
  Cable line/1(I_cable) -> I_out/1, C_cable/3(I_cable)
  Transformer-complex/1(It1) -> C_filter/2(It1)
  V_in/1 -> Cable line/1(V)
  Transformer-complex/2(It2) -> Add1/1
  Add1/1 -> C_cable/1(It2)
  Gain/1 -> Add1/2
  I_in/1 -> C_cable/2(I_in)

== system Non_WindFarm/FOM/Wind Farm/Wind Turbine Strings/String3/WT9 ==
  V_in : Inport
  I_in : Inport  Port=2
  Add1 : Sum  Inputs=+-
  C_cable : Subsystem
  C_filter : Subsystem
  Cable line : Subsystem
  Gain : Gain  Gain=1/parGrid.WTstring.Rparallel_cable
  Transformer-complex : Subsystem
  WFG : Subsystem
  V_out : Outport
  I_out : Outport  Port=2
  wires:
  I_in/1 -> C_cable/2(I_in)
  Gain/1 -> Add1/2
  Add1/1 -> C_cable/1(It2)
  Transformer-complex/2(It2) -> Add1/1
  V_in/1 -> Cable line/1(V)
  Transformer-complex/1(It1) -> C_filter/2(It1)
  Cable line/1(I_cable) -> C_cable/3(I_cable), I_out/1
  C_filter/1(Vc_filter_qd) -> Transformer-complex/1(Vc_filter_qd), WFG/1(vcqd)
  WFG/1(ilqd) -> C_filter/1(IWF)
  C_cable/1(Vc_cable) -> Cable line/2(Vc_cable), V_out/1, Transformer-complex/2(Vc_cable_qd), Gain/1

== system Non_WindFarm/FOM/Wind Farm/Wind Turbine Strings/String4/WT1 ==
  V_in : Inport
  I_in : Inport  Port=2
  Add1 : Sum  Inputs=+-
  C_cable : Subsystem
  C_filter : Subsystem
  Cable line : Subsystem
  Gain : Gain  Gain=1/parGrid.WTstring.Rparallel_cable
  Transformer-complex : Subsystem
  WFG : Subsystem
  V_out : Outport
  I_out : Outport  Port=2
  wires:
  I_in/1 -> C_cable/2(I_in)
  Gain/1 -> Add1/2
  Add1/1 -> C_cable/1(It2)
  Transformer-complex/2(It2) -> Add1/1
  V_in/1 -> Cable line/1(V)
  Transformer-complex/1(It1) -> C_filter/2(It1)
  Cable line/1(I_cable) -> C_cable/3(I_cable), I_out/1
  C_filter/1(Vc_filter_qd) -> WFG/1(vcqd), Transformer-complex/1(Vc_filter_qd)
  WFG/1(ilqd) -> C_filter/1(IWF)
  C_cable/1(Vc_cable) -> Cable line/2(Vc_cable), V_out/1, Transformer-complex/2(Vc_cable_qd), Gain/1

== system Non_WindFarm/FOM/Wind Farm/Wind Turbine Strings/String4/WT10 ==
  V_in : Inport
  I_in : Inport  Port=2
  Add1 : Sum  Inputs=+-
  C_cable : Subsystem
  C_filter : Subsystem
  Cable line : Subsystem
  Gain : Gain  Gain=1/parGrid.WTstring.Rparallel_cable
  Transformer-complex : Subsystem
  WFG : Subsystem
  V_out : Outport
  I_out : Outport  Port=2
  wires:
  C_cable/1(Vc_cable) -> Gain/1, Transformer-complex/2(Vc_cable_qd), V_out/1, Cable line/2(Vc_cable)
  WFG/1(ilqd) -> C_filter/1(IWF)
  C_filter/1(Vc_filter_qd) -> Transformer-complex/1(Vc_filter_qd), WFG/1(vcqd)
  Cable line/1(I_cable) -> I_out/1, C_cable/3(I_cable)
  Transformer-complex/1(It1) -> C_filter/2(It1)
  V_in/1 -> Cable line/1(V)
  Transformer-complex/2(It2) -> Add1/1
  Add1/1 -> C_cable/1(It2)
  Gain/1 -> Add1/2
  I_in/1 -> C_cable/2(I_in)

== system Non_WindFarm/FOM/Wind Farm/Wind Turbine Strings/String4/WT2 ==
  V_in : Inport
  I_in : Inport  Port=2
  Add1 : Sum  Inputs=+-
  C_cable : Subsystem
  C_filter : Subsystem
  Cable line : Subsystem
  Gain : Gain  Gain=1/parGrid.WTstring.Rparallel_cable
  Transformer-complex : Subsystem
  WFG : Subsystem
  V_out : Outport
  I_out : Outport  Port=2
  wires:
  C_cable/1(Vc_cable) -> Gain/1, Transformer-complex/2(Vc_cable_qd), V_out/1, Cable line/2(Vc_cable)
  WFG/1(ilqd) -> C_filter/1(IWF)
  C_filter/1(Vc_filter_qd) -> Transformer-complex/1(Vc_filter_qd), WFG/1(vcqd)
  Cable line/1(I_cable) -> I_out/1, C_cable/3(I_cable)
  Transformer-complex/1(It1) -> C_filter/2(It1)
  V_in/1 -> Cable line/1(V)
  Transformer-complex/2(It2) -> Add1/1
  Add1/1 -> C_cable/1(It2)
  Gain/1 -> Add1/2
  I_in/1 -> C_cable/2(I_in)

== system Non_WindFarm/FOM/Wind Farm/Wind Turbine Strings/String4/WT3 ==
  V_in : Inport
  I_in : Inport  Port=2
  Add1 : Sum  Inputs=+-
  C_cable : Subsystem
  C_filter : Subsystem
  Cable line : Subsystem
  Gain : Gain  Gain=1/parGrid.WTstring.Rparallel_cable
  Transformer-complex : Subsystem
  WFG : Subsystem
  V_out : Outport
  I_out : Outport  Port=2
  wires:
  I_in/1 -> C_cable/2(I_in)
  Gain/1 -> Add1/2
  Add1/1 -> C_cable/1(It2)
  Transformer-complex/2(It2) -> Add1/1
  V_in/1 -> Cable line/1(V)
  Transformer-complex/1(It1) -> C_filter/2(It1)
  Cable line/1(I_cable) -> C_cable/3(I_cable), I_out/1
  C_filter/1(Vc_filter_qd) -> Transformer-complex/1(Vc_filter_qd), WFG/1(vcqd)
  WFG/1(ilqd) -> C_filter/1(IWF)
  C_cable/1(Vc_cable) -> Cable line/2(Vc_cable), V_out/1, Transformer-complex/2(Vc_cable_qd), Gain/1

== system Non_WindFarm/FOM/Wind Farm/Wind Turbine Strings/String4/WT4 ==
  V_in : Inport
  I_in : Inport  Port=2
  Add1 : Sum  Inputs=+-
  C_cable : Subsystem
  C_filter : Subsystem
  Cable line : Subsystem
  Gain : Gain  Gain=1/parGrid.WTstring.Rparallel_cable
  Transformer-complex : Subsystem
  WFG : Subsystem
  V_out : Outport
  I_out : Outport  Port=2
  wires:
  C_cable/1(Vc_cable) -> Gain/1, Transformer-complex/2(Vc_cable_qd), V_out/1, Cable line/2(Vc_cable)
  WFG/1(ilqd) -> C_filter/1(IWF)
  C_filter/1(Vc_filter_qd) -> Transformer-complex/1(Vc_filter_qd), WFG/1(vcqd)
  Cable line/1(I_cable) -> I_out/1, C_cable/3(I_cable)
  Transformer-complex/1(It1) -> C_filter/2(It1)
  V_in/1 -> Cable line/1(V)
  Transformer-complex/2(It2) -> Add1/1
  Add1/1 -> C_cable/1(It2)
  Gain/1 -> Add1/2
  I_in/1 -> C_cable/2(I_in)

== system Non_WindFarm/FOM/Wind Farm/Wind Turbine Strings/String4/WT5 ==
  V_in : Inport
  I_in : Inport  Port=2
  Add1 : Sum  Inputs=+-
  C_cable : Subsystem
  C_filter : Subsystem
  Cable line : Subsystem
  Gain : Gain  Gain=1/parGrid.WTstring.Rparallel_cable
  Transformer-complex : Subsystem
  WFG : Subsystem
  V_out : Outport
  I_out : Outport  Port=2
  wires:
  I_in/1 -> C_cable/2(I_in)
  Gain/1 -> Add1/2
  Add1/1 -> C_cable/1(It2)
  Transformer-complex/2(It2) -> Add1/1
  V_in/1 -> Cable line/1(V)
  Transformer-complex/1(It1) -> C_filter/2(It1)
  Cable line/1(I_cable) -> C_cable/3(I_cable), I_out/1
  C_filter/1(Vc_filter_qd) -> Transformer-complex/1(Vc_filter_qd), WFG/1(vcqd)
  WFG/1(ilqd) -> C_filter/1(IWF)
  C_cable/1(Vc_cable) -> Cable line/2(Vc_cable), V_out/1, Transformer-complex/2(Vc_cable_qd), Gain/1

== system Non_WindFarm/FOM/Wind Farm/Wind Turbine Strings/String4/WT6 ==
  V_in : Inport
  I_in : Inport  Port=2
  Add1 : Sum  Inputs=+-
  C_cable : Subsystem
  C_filter : Subsystem
  Cable line : Subsystem
  Gain : Gain  Gain=1/parGrid.WTstring.Rparallel_cable
  Transformer-complex : Subsystem
  WFG : Subsystem
  V_out : Outport
  I_out : Outport  Port=2
  wires:
  C_cable/1(Vc_cable) -> Gain/1, Transformer-complex/2(Vc_cable_qd), V_out/1, Cable line/2(Vc_cable)
  WFG/1(ilqd) -> C_filter/1(IWF)
  C_filter/1(Vc_filter_qd) -> Transformer-complex/1(Vc_filter_qd), WFG/1(vcqd)
  Cable line/1(I_cable) -> I_out/1, C_cable/3(I_cable)
  Transformer-complex/1(It1) -> C_filter/2(It1)
  V_in/1 -> Cable line/1(V)
  Transformer-complex/2(It2) -> Add1/1
  Add1/1 -> C_cable/1(It2)
  Gain/1 -> Add1/2
  I_in/1 -> C_cable/2(I_in)

== system Non_WindFarm/FOM/Wind Farm/Wind Turbine Strings/String4/WT7 ==
  V_in : Inport
  I_in : Inport  Port=2
  Add1 : Sum  Inputs=+-
  C_cable : Subsystem
  C_filter : Subsystem
  Cable line : Subsystem
  Gain : Gain  Gain=1/parGrid.WTstring.Rparallel_cable
  Transformer-complex : Subsystem
  WFG : Subsystem
  V_out : Outport
  I_out : Outport  Port=2
  wires:
  I_in/1 -> C_cable/2(I_in)
  Gain/1 -> Add1/2
  Add1/1 -> C_cable/1(It2)
  Transformer-complex/2(It2) -> Add1/1
  V_in/1 -> Cable line/1(V)
  Transformer-complex/1(It1) -> C_filter/2(It1)
  Cable line/1(I_cable) -> C_cable/3(I_cable), I_out/1
  C_filter/1(Vc_filter_qd) -> Transformer-complex/1(Vc_filter_qd), WFG/1(vcqd)
  WFG/1(ilqd) -> C_filter/1(IWF)
  C_cable/1(Vc_cable) -> Cable line/2(Vc_cable), V_out/1, Transformer-complex/2(Vc_cable_qd), Gain/1

== system Non_WindFarm/FOM/Wind Farm/Wind Turbine Strings/String4/WT8 ==
  V_in : Inport
  I_in : Inport  Port=2
  Add1 : Sum  Inputs=+-
  C_cable : Subsystem
  C_filter : Subsystem
  Cable line : Subsystem
  Gain : Gain  Gain=1/parGrid.WTstring.Rparallel_cable
  Transformer-complex : Subsystem
  WFG : Subsystem
  V_out : Outport
  I_out : Outport  Port=2
  wires:
  C_cable/1(Vc_cable) -> Gain/1, Transformer-complex/2(Vc_cable_qd), V_out/1, Cable line/2(Vc_cable)
  WFG/1(ilqd) -> C_filter/1(IWF)
  C_filter/1(Vc_filter_qd) -> Transformer-complex/1(Vc_filter_qd), WFG/1(vcqd)
  Cable line/1(I_cable) -> I_out/1, C_cable/3(I_cable)
  Transformer-complex/1(It1) -> C_filter/2(It1)
  V_in/1 -> Cable line/1(V)
  Transformer-complex/2(It2) -> Add1/1
  Add1/1 -> C_cable/1(It2)
  Gain/1 -> Add1/2
  I_in/1 -> C_cable/2(I_in)

== system Non_WindFarm/FOM/Wind Farm/Wind Turbine Strings/String4/WT9 ==
  V_in : Inport
  I_in : Inport  Port=2
  Add1 : Sum  Inputs=+-
  C_cable : Subsystem
  C_filter : Subsystem
  Cable line : Subsystem
  Gain : Gain  Gain=1/parGrid.WTstring.Rparallel_cable
  Transformer-complex : Subsystem
  WFG : Subsystem
  V_out : Outport
  I_out : Outport  Port=2
  wires:
  I_in/1 -> C_cable/2(I_in)
  Gain/1 -> Add1/2
  Add1/1 -> C_cable/1(It2)
  Transformer-complex/2(It2) -> Add1/1
  V_in/1 -> Cable line/1(V)
  Transformer-complex/1(It1) -> C_filter/2(It1)
  Cable line/1(I_cable) -> C_cable/3(I_cable), I_out/1
  C_filter/1(Vc_filter_qd) -> Transformer-complex/1(Vc_filter_qd), WFG/1(vcqd)
  WFG/1(ilqd) -> C_filter/1(IWF)
  C_cable/1(Vc_cable) -> Cable line/2(Vc_cable), V_out/1, Transformer-complex/2(Vc_cable_qd), Gain/1

== system Non_WindFarm/FOM/Wind Farm/Wind Turbine Strings/String5/WT1 ==
  V_in : Inport
  I_in : Inport  Port=2
  Add1 : Sum  Inputs=+-
  C_cable : Subsystem
  C_filter : Subsystem
  Cable line : Subsystem
  Gain : Gain  Gain=1/parGrid.WTstring.Rparallel_cable
  Transformer-complex : Subsystem
  WFG : Subsystem
  V_out : Outport
  I_out : Outport  Port=2
  wires:
  I_in/1 -> C_cable/2(I_in)
  Gain/1 -> Add1/2
  Add1/1 -> C_cable/1(It2)
  Transformer-complex/2(It2) -> Add1/1
  V_in/1 -> Cable line/1(V)
  Transformer-complex/1(It1) -> C_filter/2(It1)
  Cable line/1(I_cable) -> C_cable/3(I_cable), I_out/1
  C_filter/1(Vc_filter_qd) -> WFG/1(vcqd), Transformer-complex/1(Vc_filter_qd)
  WFG/1(ilqd) -> C_filter/1(IWF)
  C_cable/1(Vc_cable) -> Cable line/2(Vc_cable), V_out/1, Transformer-complex/2(Vc_cable_qd), Gain/1
